simulink model "engine_idle_speed"  (Simulink 6.0)
settings: Solver=ode45  StartTime=0  StopTime=150  RelTol=1e-3
PreLoadFcn:
  | load engine_idle_speed
values from neighbouring files (symbols this model uses):
  damp1 = 0.707    [engine_idle_speed.mat]    (also in engine_sweep.mat; iodataval.mat)
  damp2 = 0.707    [engine_idle_speed.mat]    (also in engine_sweep.mat; iodataval.mat)
  damp3 = 0.707    [engine_idle_speed.mat]    (also in engine_sweep.mat; iodataval.mat)
  delay = 0.0001    [engine_idle_speed.mat]    (also in engine_sweep.mat; iodataval.mat)
  freq1 = 3    [engine_idle_speed.mat]    (also in engine_sweep.mat; iodataval.mat)
  freq2 = 3    [engine_idle_speed.mat]    (also in engine_sweep.mat; iodataval.mat)
  freq3 = 3    [engine_idle_speed.mat]    (also in engine_sweep.mat; iodataval.mat)
  gain1 = 100    [engine_idle_speed.mat]    (also in engine_sweep.mat; iodataval.mat)
  gain2 = 0    [engine_idle_speed.mat]    (also in engine_sweep.mat; iodataval.mat)
  gain3 = 0    [engine_idle_speed.mat]    (also in engine_sweep.mat; iodataval.mat)
  mean_speed = 600    [engine_idle_speed.mat]    (also in engine_sweep.mat; iodataval.mat)
settings Model: Creator=beryilma  LastModifiedBy=beryilma
settings DataIOCC: LimitDataPoints=off  SaveOutput=off  SaveTime=off  SignalLoggingName=logsOut
settings OptimizationCC: BooleanDataType=off
settings DebuggingCC: CheckExecutionContextPreStartOutputMsg=on  CheckExecutionContextRuntimeOutputMsg=on  SolverPrmCheckMsg=none
settings HardwareCC: TargetUnknown=on
settings ModelReferenceCC: UpdateModelReferenceTargets=IfOutOfDate
settings RTWCC: ProfileTLC=on
settings GRTTargetCC: LifeSpan=inf
settings SFSimCC: SFSimApplyToAllLibs=on  SFSimBuildMode=Incremental

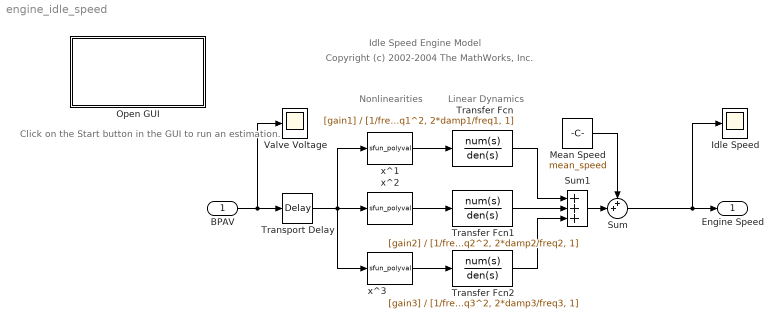
== system engine_idle_speed ==
  note: Idle Speed Engine Model
  note: Nonlinearities
  note: Copyright (c) 2002-2004 The MathWorks, Inc.
  note: Linear Dynamics
  note: Click on the Start button in the GUI to
      | run an estimation.
  BPAV : Inport  LatchInput=off
  Idle Speed : Scope
      settings: TickLabels=on  TimeRange=150  YMin=600  YMax=950  DataFormat=Array
  Mean Speed : Constant  Value=mean_speed
  Open GUI : Subsystem  EnableExecutionContextPropagation=on
      settings: OpenFcn=|
      | [F,W,M] = slctrlexplorer('initialize');
      | p = M.load('engine_idle_speed_project');
      | W.addNode(p);
      | h = find(p, '-class', 'spenodes.EstimationLeaf');
      | F.setSelected(h.getTreeNodeInterface);
      | drawnow;
      | runpanel = h.getDialogInterface(M).getEstimationRun;
      | tabpanel = runpanel.getParent;
      | awtinvoke(tabpanel, 'setSelectedComponent', runpanel);
      | F.setVisible(1);
      mask Display: disp('Double click here\nto open\nParameter Estimation\nGUI with preload data')
  Sum : Sum  Inputs=++|
  Sum1 : Sum  Inputs=+++
  Transfer Fcn : TransferFcn  Numerator=[gain1]  Denominator=[1/freq1^2, 2*damp1/freq1, 1]
  Transfer Fcn1 : TransferFcn  Numerator=[gain2]  Denominator=[1/freq2^2, 2*damp2/freq2, 1]
  Transfer Fcn2 : TransferFcn  Numerator=[gain3]  Denominator=[1/freq3^2, 2*damp3/freq3, 1]
  Transport Delay : TransportDelay  DelayTime=delay  PadeOrder=1
  Valve Voltage : Scope
      settings: TickLabels=on  TimeRange=150  YMin=-1.5  YMax=1.5  DataFormat=Array
  x^1 : S-Function  AncestorBlock=simulink/Math Operations/Polynomial  FunctionName=sfun_polyval  Parameters=coefs  mask(Polyval){coefs=[1 0]}
      mask prompts: coefs "Polynomial coefficients:"
      mask help: Polynomial evaluation. Calculates P(u) given by the polynomial coefficient array P. P is sorted highest order to lowest order, the form accepted by MATLAB's polyval function.
      mask init:
      | if isempty(coefs)
      |   str = 'O(P) = ???';
      | else
      |   str = sprintf('O(P) = %d',length(coefs)-1);
      | end
      mask Display: text(0.35,0.5, 'x^1')
  x^2 : S-Function  AncestorBlock=simulink/Math Operations/Polynomial  FunctionName=sfun_polyval  Parameters=coefs  mask(Polyval){coefs=[1 0 0]}
      mask prompts: coefs "Polynomial coefficients:"
      mask help: Polynomial evaluation. Calculates P(u) given by the polynomial coefficient array P. P is sorted highest order to lowest order, the form accepted by MATLAB's polyval function.
      mask init:
      | if isempty(coefs)
      |   str = 'O(P) = ???';
      | else
      |   str = sprintf('O(P) = %d',length(coefs)-1);
      | end
      mask Display: text(0.35,0.5, 'x^2')
  x^3 : S-Function  AncestorBlock=simulink/Math Operations/Polynomial  FunctionName=sfun_polyval  Parameters=coefs  mask(Polyval){coefs=[1 0 0 0]}
      mask prompts: coefs "Polynomial coefficients:"
      mask help: Polynomial evaluation. Calculates P(u) given by the polynomial coefficient array P. P is sorted highest order to lowest order, the form accepted by MATLAB's polyval function.
      mask init:
      | if isempty(coefs)
      |   str = 'O(P) = ???';
      | else
      |   str = sprintf('O(P) = %d',length(coefs)-1);
      | end
      mask Display: text(0.35,0.5, 'x^3')
  Engine Speed : Outport
  wires:
  BPAV/1 -> Transport Delay/1, Valve Voltage/1
  Transfer Fcn/1 -> Sum1/1
  Transfer Fcn1/1 -> Sum1/2
  Transfer Fcn2/1 -> Sum1/3
  x^1/1 -> Transfer Fcn/1
  x^3/1 -> Transfer Fcn2/1
  x^2/1 -> Transfer Fcn1/1
  Transport Delay/1 -> x^2/1, x^1/1, x^3/1
  Sum1/1 -> Sum/2
  Mean Speed/1 -> Sum/1
  Sum/1 -> Engine Speed/1, Idle Speed/1

== system engine_idle_speed/Open GUI ==
